simulink model "Force_control_24"  (R2024b)
settings: Solver=VariableStepAuto  StartTime=0.0  StopTime=20  RelTol=1e-3
values from neighbouring files (symbols this model uses):
  f_d = [10; 0]    [config_robot.m]
  K = [1000, 0 ... (first row only)    [config_robot.m]
  K_D = [5000, 0 ... (first row only)    [config_robot.m]
  K_F = [0.03, 0 ... (first row only)    [config_robot.m]
  K_I = [0.03, 0 ... (first row only)    [config_robot.m]
  K_P = [5000, 0 ... (first row only)    [config_robot.m]
  x_e_initial = [1.3; 0.7]    [config_robot.m]
  x_r = [1.2; 0.7]    [config_robot.m]
undefined symbols (not defined in the file or in its folder): C_F, M_d_inv
settings Model: Creator=Johannes  LastModifiedBy=Usuario
settings ConfigComp: CovBoundaryAbsTol=1.0e-5

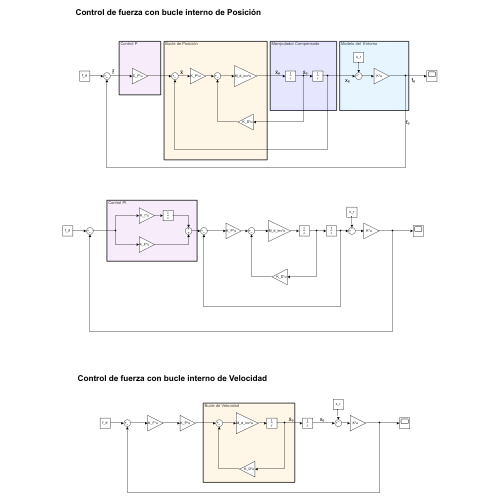
[thumbnail: Simulink's stored preview of the top-level diagram]
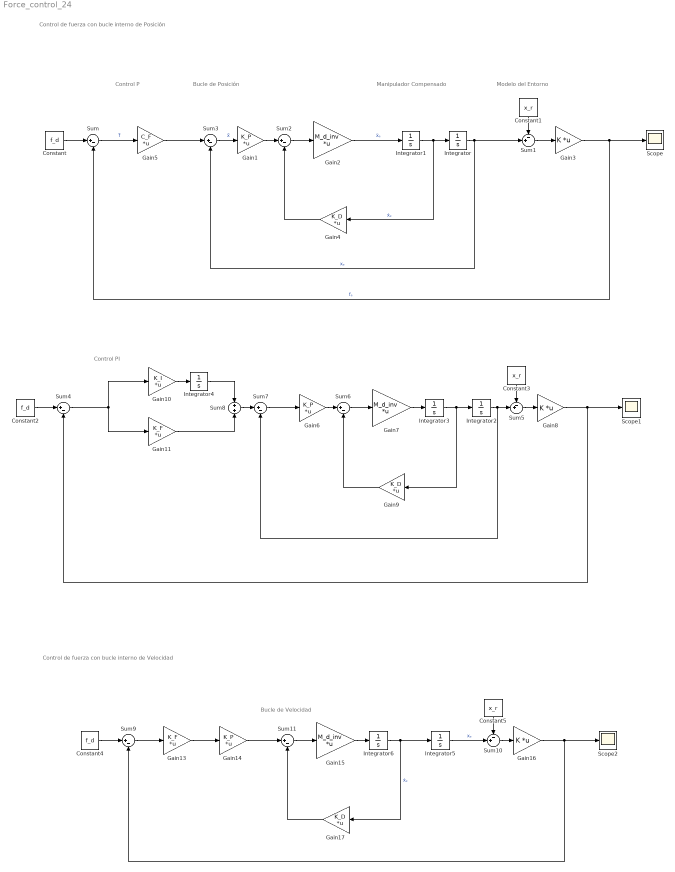
== system Force_control_24 ==
  note: Control de fuerza con bucle interno de Posición
  note: Control PI
  note: Modelo del Entorno
  note: Manipulador Compensado
  note: Bucle de Posición
  note: Control P
  note: Bucle de Velocidad
  note: Control de fuerza con bucle interno de Velocidad
  Constant : Constant  Value=f_d
  Constant1 : Constant  Value=x_r
  Constant2 : Constant  Value=f_d
  Constant3 : Constant  Value=x_r
  Constant4 : Constant  Value=f_d
  Constant5 : Constant  Value=x_r
  Gain1 : Gain  Gain=K_P  Multiplication=Matrix(K*u)
  Gain10 : Gain  Gain=K_I  Multiplication=Matrix(K*u)
  Gain11 : Gain  Gain=K_F  Multiplication=Matrix(K*u)
  Gain13 : Gain  Gain=K_F  Multiplication=Matrix(K*u)
  Gain14 : Gain  Gain=K_P  Multiplication=Matrix(K*u)
  Gain15 : Gain  Gain=M_d_inv  Multiplication=Matrix(K*u)
  Gain16 : Gain  Gain=K  Multiplication=Matrix(K*u)
  Gain17 : Gain  Gain=K_D  Multiplication=Matrix(K*u)
  Gain2 : Gain  Gain=M_d_inv  Multiplication=Matrix(K*u)
  Gain3 : Gain  Gain=K  Multiplication=Matrix(K*u)
  Gain4 : Gain  Gain=K_D  Multiplication=Matrix(K*u)
  Gain5 : Gain  Gain=C_F  Multiplication=Matrix(K*u)
  Gain6 : Gain  Gain=K_P  Multiplication=Matrix(K*u)
  Gain7 : Gain  Gain=M_d_inv  Multiplication=Matrix(K*u)
  Gain8 : Gain  Gain=K  Multiplication=Matrix(K*u)
  Gain9 : Gain  Gain=K_D  Multiplication=Matrix(K*u)
  Integrator : Integrator  InitialCondition=x_e_initial
  Integrator{1,3..4,6} (4 alike) : Integrator
  Integrator2 : Integrator  InitialCondition=x_e_initial
  Integrator5 : Integrator  InitialCondition=x_e_initial
  Scope : Scope
  Scope1 : Scope
  Scope2 : Scope
  Sum{,2..4,6..7,9,11} (8 alike) : Sum  Inputs=|+-
  Sum1 : Sum  Inputs=-+|
  Sum10 : Sum  Inputs=-+|
  Sum5 : Sum  Inputs=-+|
  Sum8 : Sum  Inputs=+|+
  wires:
  Gain5/1 -> Sum3/1
  Gain1/1 -> Sum2/1
  Sum/1 -> Gain5/1  "f̃"
  Constant/1 -> Sum/1
  Integrator1/1 -> Integrator/1, Gain4/1  "ẋₑ"
  Integrator/1 -> Sum1/2, Sum3/2  "xₑ"
  Sum3/1 -> Gain1/1  "x̃"
  Sum2/1 -> Gain2/1
  Gain2/1 -> Integrator1/1  "ẍₑ"
  Gain4/1 -> Sum2/2
  Gain3/1 -> Scope/1, Sum/2  "fₑ"
  Sum1/1 -> Gain3/1
  Constant1/1 -> Sum1/1
  Gain6/1 -> Sum6/1
  Gain9/1 -> Sum6/2
  Constant3/1 -> Sum5/1
  Sum4/1 -> Gain11/1, Gain10/1
  Gain7/1 -> Integrator3/1
  Sum5/1 -> Gain8/1
  Gain8/1 -> Scope1/1, Sum4/2
  Constant2/1 -> Sum4/1
  Integrator3/1 -> Integrator2/1, Gain9/1
  Sum7/1 -> Gain6/1
  Integrator2/1 -> Sum5/2, Sum7/2
  Sum8/1 -> Sum7/1
  Sum6/1 -> Gain7/1
  Gain10/1 -> Integrator4/1
  Integrator4/1 -> Sum8/1
  Gain11/1 -> Sum8/2
  Gain13/1 -> Gain14/1
  Integrator6/1 -> Integrator5/1, Gain17/1  "ẋₑ"
  Gain16/1 -> Scope2/1, Sum9/2
  Sum11/1 -> Gain15/1
  Gain15/1 -> Integrator6/1
  Gain17/1 -> Sum11/2
  Gain14/1 -> Sum11/1
  Sum10/1 -> Gain16/1
  Constant4/1 -> Sum9/1
  Integrator5/1 -> Sum10/2  "xₑ"
  Constant5/1 -> Sum10/1
  Sum9/1 -> Gain13/1
